simulink model "CEGR_Vehicle_10kW_GZS60_v03_stage2_steadyfit"  (R2025b)
settings: Solver=FixedStepDiscrete  StartTime=0.0  StopTime=120  FixedStep=0.1  RelTol=1e-3
model workspace (MAT data in the model file):
  CompressorParam_v2 = [55; 35]
  EGRInitialNode_v2 = [0; 0; 0; 0; 25; 101.325; 0]
  EnvParam_v2 = [96485.33212; 0.031998; 0.0280134; 0.01801528; 101.325; 25; 0.5; 0.2095; 0.7905; 16; 2]
  HumidifierParam_v2 = [0.031998; 0.0280134; 0.01801528; 101.325; 55; 0.47854; 0.0983333333333; 0.37998; 0.5825; 4.58289; 11.4663; 0.868128; 40; 5e-05; 1e-09; 0.02; 0.02; 80]
  I_stack_cmd_A = 120
  IntercoolerParam_v2 = [0.031998; 0.0280134; 0.01801528; 101.325; 55; 8]
  P_v2.rootDir = 'E:\agentwork_pemfc_cEGR_0519\01_自吸方案\01_车载系统_10kW_GZS60_v3'
  P_v2.inputDir = 'E:\agentwork_pemfc_cEGR_0519\01_自吸方案\01_车载系统_10kW_GZS60_v3\00_输入参数'
  P_v2.modelName = 'CEGR_Vehicle_10kW_GZS60_v03'
  P_v2.modelFile = 'E:\agentwork_pemfc_cEGR_0519\01_自吸方案\01_车载系统_10kW_GZS60_v3\01_模型\CEGR_Vehicle_10kW_GZS60_v03.slx'
  P_v2.stopTime_s = 120
  P_v2.dt_s = 0.1
  P_v2.R_J_molK = 8.314462618
  P_v2.F_C_mol = 96485.33212
  P_v2.M_O2_kg_mol = 0.031998
  P_v2.M_N2_kg_mol = 0.0280134
  P_v2.M_H2O_kg_mol = 0.01801528
  P_v2.M_H2_kg_mol = 0.00201588
  P_v2.p_amb_kPa = 101.325
  P_v2.T_amb_C = 25
  P_v2.RH_amb = 0.5
  P_v2.xO2_dry = 0.2095
  P_v2.xN2_dry = 0.7905
  P_v2.N_cell = 16
  P_v2.A_cell_cm2 = 380
  P_v2.I_stack_default_A = 120
  P_v2.oxygen_stoich = 2
  P_v2.anode_stoich = 1.35
  P_v2.RH_an_in = 0.3
  P_v2.compressor_dp_kPa = 55
  P_v2.compressor_dT_C = 35
  P_v2.intercooler_T_C = 55
  P_v2.intercooler_dp_kPa = 8
  P_v2.p_cathode_back_kPa = 128
  P_v2.p_anode_back_kPa = 85
  P_v2.p_anode_in_kPa = 140
  P_v2.K_ca_in_kg_s_kPa = 0.00135
  P_v2.hum_NTU_ref = 0.47854
  P_v2.hum_m_ref_kg_s = 0.0983333333333
  P_v2.hum_flow_exp = 0.37998
  P_v2.hum_heat_eff = 0.5825
  P_v2.hum_dry_dp_ref_kPa = 4.58289
  P_v2.hum_wet_dp_ref_kPa = 11.4663
  P_v2.hum_dp_exp = 0.868128
  P_v2.hum_mem_area_m2 = 40
  P_v2.hum_mem_thickness_m = 5e-05
  P_v2.hum_mem_D_eff_m2_s = 1e-09
  P_v2.hum_beta_wet_m_s = 0.02
  P_v2.hum_beta_dry_m_s = 0.02
  P_v2.hum_UA_W_K = 80
  P_v2.V_ca_m3 = 0.0025
  P_v2.V_an_m3 = 0.0012
  P_v2.K_ca_out_kg_s_kPa = 0.000216
  P_v2.K_an_out_kg_s_kPa = 6.67e-06
  P_v2.K_liq_carry_1_s = 0.08
  P_v2.C_stack_J_K = 45000
  P_v2.h_cool_W_K = 121
  P_v2.T_cool_C = 62
  P_v2.h_amb_W_K = 9
  P_v2.k_mem_water_kg_s = 0.00012
  P_v2.E_nernst_ref_V = 1.229
  P_v2.E_nernst_temp_coeff_V_K = 0.000845879868025
  P_v2.book_xi1 = -1.18256193785
  P_v2.book_xi2 = 0.00294108739023
  P_v2.book_xi3 = 5.21269240296e-05
  P_v2.book_xi4 = -8.54349163446e-05
  P_v2.membraneThickness_cm = 0.005
  P_v2.book_contact_resistance_ohm = 2.22044867148e-14
  P_v2.book_concentration_m_V = 3.97280101898e-05
  P_v2.book_concentration_n_1_A = 0.00982352283961
  P_v2.thermoneutralVoltage_V = 1.254
  P_v2.LHV_H2_J_mol = 241800
  P_v2.stack_m_act_O2 = 0.65
  P_v2.stack_m_lim_O2 = 1.2
  P_v2.stack_i_lim_ref_A_cm2 = 1.2
  P_v2.stack_lambda_O2_half = 1.2
  P_v2.separator_liq_eff = 0.98
  P_v2.egr_fraction_default = 0.4
  P_v2.separator_dp_ref_kPa = 2
  P_v2.tailgas_manifold_dp_kPa = 0.5
  P_v2.egr_return_target_margin_kPa = 0
  P_v2.V_tailgas_manifold_m3 = 0.003
  P_v2.K_tailgas_egr_out_kg_s_kPa = 4e-05
  P_v2.K_tailgas_bp_out_kg_s_kPa = 0.00012
  P_v2.egr_valve_coeff = 1.2
  P_v2.egr_valve_dp_fraction = 0.65
  P_v2.bp_valve_coeff = 2.8
  P_v2.egr_return_pipe_dp_ref_kPa = 1.5
  P_v2.egr_return_pipe_dp_exp = 1
  P_v2.p_anode_tail_downstream_kPa = 85
  P_v2.V_ca_manifold_m3 = 0.0011
  P_v2.V_an_manifold_m3 = 0.0032
  P_v2.K_ca_man_out_kg_s_kPa = 0.0012
  P_v2.K_an_man_out_kg_s_kPa = 4e-05
  P_v2.EnvParam = [96485.33212; 0.031998; 0.0280134; 0.01801528; 101.325; 25; 0.5; 0.2095; 0.7905; 16; 2]
  P_v2.CompressorParam = [55; 35]
  P_v2.IntercoolerParam = [0.031998; 0.0280134; 0.01801528; 101.325; 55; 8]
  P_v2.HumidifierParam = [0.031998; 0.0280134; 0.01801528; 101.325; 55; 0.47854; 0.0983333333333; 0.37998; 0.5825; 4.58289; 11.4663; 0.868128; 40; 5e-05; 1e-09; 0.02; 0.02; 80]
  P_v2.StackParam = [8.314462618; 96485.33212; 0.031998; 0.0280134; 0.01801528; 0.00201588; 101.325; 25; 16; 380; 0.0025; 0.0012; 0.000216; 6.67e-06; 128; 85; 0.08; 45000; 121; 62; 9; 1.229; 0.000845879868025; -1.18256193785; 0.00294108739023; 5.21269240296e-05; -8.54349163446e-05; 0.005; 2.22044867148e-14; 3.97280101898e-05; 0.00982352283961; 1.254; 1.35; 0.3; 0.1; 0.00012; 140; 0.00135; 0.65; 1.2; 1.2; 1.2; 241800]
  P_v2.SeparatorParam = [0.031998; 0.0280134; 0.01801528; 0.98; 101.325; 2; 0.0983333333333; 0.72344]
  P_v2.TailGasParam = [8.314462618; 0.031998; 0.0280134; 0.01801528; 0.003; 4e-05; 0.00012; 0.08; 0.1; 101.325; 0]
  P_v2.CathodeOutletManifoldParam = [8.314462618; 0.031998; 0.0280134; 0.01801528; 0.0011; 0.0012; 0.08; 0.1; 101.325]
  P_v2.AnodeOutletManifoldParam = [8.314462618; 0.00201588; 0.0280134; 0.01801528; 0.0032; 4e-05; 0.08; 0.1; 101.325]
  P_v2.EGRValveParam = [1.2; 0.65]
  P_v2.BackPressureValveParam = [2.8; 101.325]
  P_v2.EGRReturnPipeParam = [101.325; 1.5; 0.0983333333333; 1]
  P_v2.egr_initial_node = [0; 0; 0; 0; 25; 101.325; 0]
  P_v2.wet_initial_node = [0; 0; 0; 0; 70; 128; 0]
  P_v2.ca_manifold_initial_state = [0.000232010722367; 0.000925320943558; 0.00017649999609; 0]
  P_v2.an_manifold_initial_state = [0.000177788459184; 0; 0.000154036360224; 0]
  P_v2.tailgas_manifold_initial_state = [0.000549996359197; 0.00219353288871; 0.0004813636257; 0]
  P_v2.stack_initial_state = [0.000711310590109; 0.00236638748431; 0.000400476887549; 0; 0.000111852500588; 5.7763635084e-05; 0; 65]
  P_v2.stack_initial_state_audit = [0.000711310590109; 0.00236638748431; 0.000400476887549; 0.000111852500588; 5.7763635084e-05; 65]
  StackInitialStateAudit_v3 = [0.000711310590109; 0.00236638748431; 0.000400476887549; 0.000111852500588; 5.7763635084e-05; 65]
  StackParam_v2 = [8.314462618; 96485.33212; 0.031998; 0.0280134; 0.01801528; 0.00201588; 101.325; 25; 16; 380; 0.0025; 0.0012; 0.000216; 6.67e-06; 128; 85; 0.08; 45000; 121; 62; 9; 1.229; 0.000845879868025; -1.18256193785; 0.00294108739023; 5.21269240296e-05; -8.54349163446e-05; 0.005; 2.22044867148e-14; 3.97280101898e-05; 0.00982352283961; 1.254; 1.35; 0.3; 0.1; 0.00012; 140; 0.00135; 0.65; 1.2; 1.2; 1.2; 241800]
  WetInitialNode_v2 = [0; 0; 0; 0; 70; 128; 0]
  egr_fraction_cmd = 0
settings Model: Creator=ADMIN  LastModifiedBy=ADMIN

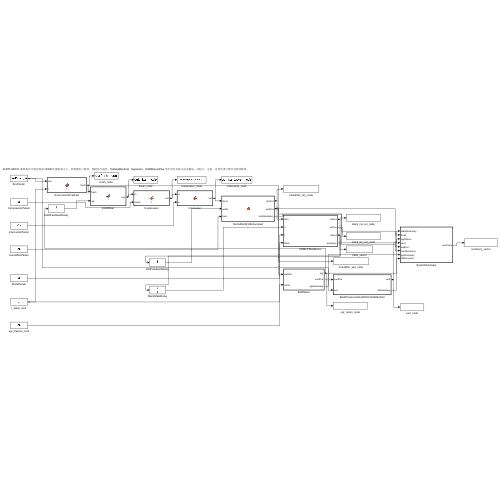
[thumbnail: Simulink's stored preview of the top-level diagram]
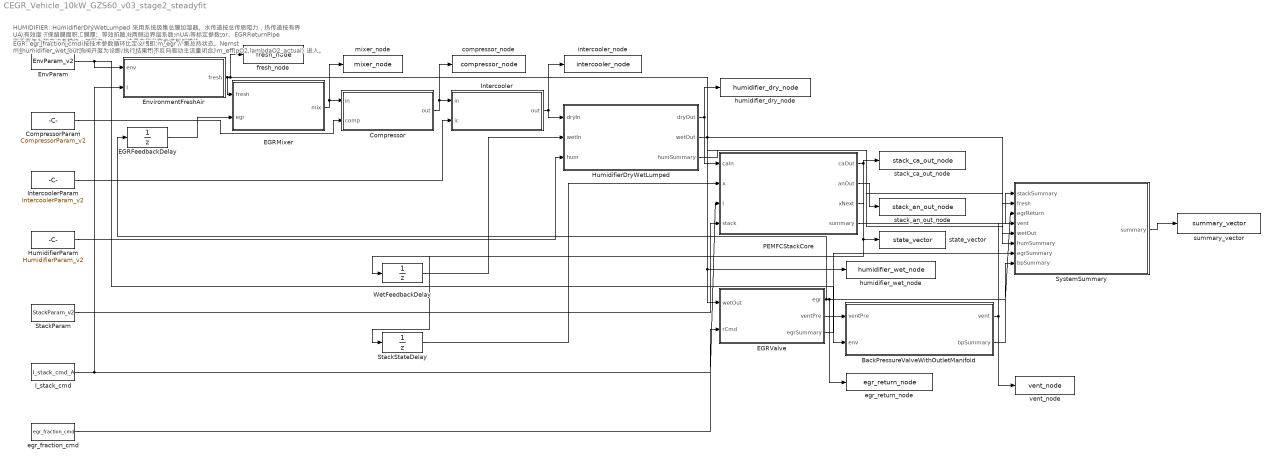
== system CEGR_Vehicle_10kW_GZS60_v03_stage2_steadyfit ==
  note: AUDIT-ARCH: 新架构审计版仅保留 cEGR 性能影响主干。旧阴极出口歧管、阳极尾气歧管、TailGasManifold、Separator、EGRReturnPipe 等不再作为独立动态模块；其阻力、分流、边界作用已整合进相邻模块。
  note: STACK: PEMFCStackCore 使用 5 个气体组分质量状态 + 1 个集总热状态。Nernst 不做经验修改，氧浓度影响通过活化过电势 i0_c_eff(pO2) 和浓差过电势 i_lim_eff(pO2,lambdaO2_actual) 进入。
  note: HUMIDIFIER: HumidifierDryWetLumped 采用系统级集总膜加湿器。水传递按总传质阻力，热传递按有界 UA/有效度，保留膜面积、膜厚、等效扩散、两侧边界层系数、UA 等标定参数。
  note: EGR: egr_fraction_cmd 按技术参数循环比定义，即 m_egr / m_humidifier_wet_out。阀开度为诊断/执行结果，不反向驱动主流量闭合。
  BackPressureValveWithOutletManifold : MATLAB Function  TreatAsAtomicUnit=on
  Compressor : MATLAB Function  TreatAsAtomicUnit=on
  CompressorParam : Constant  Value=CompressorParam_v2
  EGRFeedbackDelay : UnitDelay  InitialCondition=EGRInitialNode_v2  SampleTime=-1  HasFrameUpgradeWarning=on
  EGRMixer : MATLAB Function  TreatAsAtomicUnit=on
  EGRValve : MATLAB Function  TreatAsAtomicUnit=on
  EnvParam : Constant  Value=EnvParam_v2
  EnvironmentFreshAir : MATLAB Function  TreatAsAtomicUnit=on
  HumidifierDryWetLumped : MATLAB Function  TreatAsAtomicUnit=on
  HumidifierParam : Constant  Value=HumidifierParam_v2
  I_stack_cmd : Constant  Value=I_stack_cmd_A
  Intercooler : MATLAB Function  TreatAsAtomicUnit=on
  IntercoolerParam : Constant  Value=IntercoolerParam_v2
  PEMFCStackCore : MATLAB Function  TreatAsAtomicUnit=on
  StackParam : Constant  Value=StackParam_v2
  StackStateDelay : UnitDelay  InitialCondition=StackInitialStateAudit_v3  SampleTime=-1  HasFrameUpgradeWarning=on
  SystemSummary : MATLAB Function  TreatAsAtomicUnit=on
  WetFeedbackDelay : UnitDelay  InitialCondition=WetInitialNode_v2  SampleTime=-1  HasFrameUpgradeWarning=on
  compressor_node : ToWorkspace  VariableName=compressor_node  SampleTime=-1
  egr_fraction_cmd : Constant  Value=egr_fraction_cmd
  egr_return_node : ToWorkspace  VariableName=egr_return_node  SampleTime=-1
  fresh_node : ToWorkspace  VariableName=fresh_node  SampleTime=-1
  humidifier_dry_node : ToWorkspace  VariableName=humidifier_dry_node  SampleTime=-1
  humidifier_wet_node : ToWorkspace  VariableName=humidifier_wet_node  SampleTime=-1
  intercooler_node : ToWorkspace  VariableName=intercooler_node  SampleTime=-1
  mixer_node : ToWorkspace  VariableName=mixer_node  SampleTime=-1
  stack_an_out_node : ToWorkspace  VariableName=stack_an_out_node  SampleTime=-1
  stack_ca_out_node : ToWorkspace  VariableName=stack_ca_out_node  SampleTime=-1
  state_vector : ToWorkspace  VariableName=state_vector  SampleTime=-1
  summary_vector : ToWorkspace  VariableName=summary_vector  SampleTime=-1
  vent_node : ToWorkspace  VariableName=vent_node  SampleTime=-1
  wires:
  EnvParam/1 -> EnvironmentFreshAir/1(env), BackPressureValveWithOutletManifold/2(env)
  I_stack_cmd/1 -> EnvironmentFreshAir/2(I), PEMFCStackCore/3(I)
  EnvironmentFreshAir/1(fresh) -> fresh_node/1, SystemSummary/2(fresh), EGRMixer/1(fresh)
  EGRFeedbackDelay/1 -> EGRMixer/2(egr)
  EGRMixer/1(mix) -> Compressor/1(in), mixer_node/1
  CompressorParam/1 -> Compressor/2(comp)
  Compressor/1(out) -> Intercooler/1(in), compressor_node/1
  IntercoolerParam/1 -> Intercooler/2(ic)
  Intercooler/1(out) -> HumidifierDryWetLumped/1(dryIn), intercooler_node/1
  WetFeedbackDelay/1 -> HumidifierDryWetLumped/2(wetIn)
  HumidifierParam/1 -> HumidifierDryWetLumped/3(hum)
  HumidifierDryWetLumped/1(dryOut) -> PEMFCStackCore/1(caIn), humidifier_dry_node/1
  StackStateDelay/1 -> PEMFCStackCore/2(x)
  StackParam/1 -> PEMFCStackCore/4(stack)
  PEMFCStackCore/1(caOut) -> WetFeedbackDelay/1, stack_ca_out_node/1
  PEMFCStackCore/2(anOut) -> stack_an_out_node/1
  PEMFCStackCore/3(xNext) -> StackStateDelay/1, state_vector/1
  HumidifierDryWetLumped/2(wetOut) -> EGRValve/1(wetOut), humidifier_wet_node/1, SystemSummary/5(wetOut)
  egr_fraction_cmd/1 -> EGRValve/2(rCmd)
  EGRValve/1(egr) -> egr_return_node/1, SystemSummary/3(egrReturn), EGRFeedbackDelay/1
  EGRValve/2(ventPre) -> BackPressureValveWithOutletManifold/1(ventPre)
  BackPressureValveWithOutletManifold/1(vent) -> vent_node/1, SystemSummary/4(vent)
  PEMFCStackCore/4(summary) -> SystemSummary/1(stackSummary)
  HumidifierDryWetLumped/3(humSummary) -> SystemSummary/6(humSummary)
  EGRValve/3(egrSummary) -> SystemSummary/7(egrSummary)
  BackPressureValveWithOutletManifold/2(bpSummary) -> SystemSummary/8(bpSummary)
  SystemSummary/1(summary) -> summary_vector/1

== matlab function CEGR_Vehicle_10kW_GZS60_v03_stage2_steadyfit/EGRMixer ==
  data: fresh input; mix output; egr input
function mix = f(fresh, egr)
%#codegen
% EGR 掺混口径：总进空压机质量流保持新鲜空气基准，回流尾气替代等质量新鲜空气。
mix=zeros(7,1); mf0=max(sum(fresh(1:4)),0); me0=max(sum(egr(1:4)),0); me=min(me0,0.95*mf0); mf=max(mf0-me,0);
wFresh=fresh(1:4)/max(mf0,1e-12); wEgr=egr(1:4)/max(me0,1e-12);
mix(1:4)=mf*wFresh+me*wEgr; mt=max(mf+me,1e-12);
mix(5)=(fresh(5)*mf+egr(5)*me)/mt;
mix(6)=(fresh(6)*mf+egr(6)*me)/mt;
mix(7)=double(mix(4)>1e-12);
end

== matlab function CEGR_Vehicle_10kW_GZS60_v03_stage2_steadyfit/EnvironmentFreshAir ==
  data: env input; fresh output; I input
function fresh = f(env, I)
%#codegen
F=env(1); M_O2=env(2); M_N2=env(3); M_H2O=env(4); pamb=env(5); Tamb=env(6); RH=env(7); xO2=env(8); xN2=env(9); N=env(10); stoich=env(11);
psat=sat_kPa(Tamb); pH2O=min(RH*psat,0.98*pamb); pdry=max(pamb-pH2O,1e-6);
pO2=xO2*pdry; pN2=xN2*pdry;
nO2=stoich*max(I,0)*N/(4*F);
mO2=max(nO2*M_O2,1e-7); scale=(mO2/M_O2)/max(pO2,1e-9);
fresh=[mO2; pN2*scale*M_N2; pH2O*scale*M_H2O; 0; Tamb; pamb; 0];
end
function p=sat_kPa(T)
p=0.61121*exp((18.678-T/234.5)*(T/(257.14+T)));
end

== matlab function CEGR_Vehicle_10kW_GZS60_v03_stage2_steadyfit/Compressor ==
  data: in input; out output; comp input
function out = f(in, comp)
%#codegen
out=in; out(6)=in(6)+comp(1); out(5)=in(5)+comp(2); out(7)=double(out(4)>1e-12);
end

== matlab function CEGR_Vehicle_10kW_GZS60_v03_stage2_steadyfit/Intercooler ==
  data: in input; out output; ic input
function out = f(in, ic)
%#codegen
out=in; M_O2=ic(1); M_N2=ic(2); M_H2O=ic(3); pamb=ic(4); Tout=ic(5); dp=ic(6);
out(5)=Tout; out(6)=max(in(6)-dp,pamb);
ps=min(sat_kPa(Tout),0.98*out(6)); nDry=max(out(1)/M_O2+out(2)/M_N2,1e-12); mSat=ps*nDry/max(out(6)-ps,1e-6)*M_H2O;
if out(3)>mSat, out(4)=out(4)+out(3)-mSat; out(3)=mSat; end
out(7)=double(out(4)>1e-12);
end
function p=sat_kPa(T)
p=0.61121*exp((18.678-T/234.5)*(T/(257.14+T)));
end

== matlab function CEGR_Vehicle_10kW_GZS60_v03_stage2_steadyfit/HumidifierDryWetLumped ==
  data: dryIn input; dryOut output; wetIn input; hum input; wetOut output; humSummary output
function [dryOut, wetOut, humSummary] = f(dryIn, wetIn, hum)
%#codegen
M_O2=hum(1); M_N2=hum(2); M_H2O=hum(3); pamb=hum(4); mRef=max(hum(7),1e-9);
A=hum(13); delta=max(hum(14),1e-9); Deff=max(hum(15),1e-12); betaW=max(hum(16),1e-6); betaD=max(hum(17),1e-6); UA=max(hum(18),0);
mDry=max(sum(dryIn(1:4)),1e-9); mWet=max(sum(wetIn(1:4)),1e-9);
pD=vapor_p(dryIn,M_O2,M_N2,M_H2O); pW=vapor_p(wetIn,M_O2,M_N2,M_H2O);
Rtot=1/betaW+delta/Deff+1/betaD;
j=max((pW-pD)*1000,0)/(8.314462618*max(dryIn(5)+273.15,250)*Rtot);
mTransRaw=j*A*M_H2O; dryNeed=max(vapor_sat_mass(dryIn(1),dryIn(2),dryIn(5),dryIn(6),hum)-dryIn(3),0); wetAvail=max(wetIn(3),0);
mTrans=min([mTransRaw,dryNeed,wetAvail]);
Cmin=max(min(mDry,mWet)*1050,1e-6); epsH=min(max(1-exp(-UA/Cmin),0),0.85); dTDry=min(max(epsH*(wetIn(5)-dryIn(5))*Cmin/(mDry*1050),-30),30);
dryOut=dryIn; dryOut(3)=dryIn(3)+mTrans; dryOut(5)=min(max(dryIn(5)+dTDry,-20),95);
dpDry=hum(10)*(mDry/mRef)^hum(12); dryOut(6)=max(dryIn(6)-dpDry,pamb);
[dryOut(3),dryOut(4)]=clip_vapor(dryOut(3),dryOut(4),dryOut(1),dryOut(2),dryOut(5),dryOut(6),hum); dryOut(7)=double(dryOut(4)>1e-12);
wetOut=wetIn; wetOut(3)=max(wetIn(3)-mTrans,0); wetOut(5)=min(max(wetIn(5)-dTDry,-20),95);
dpWet=hum(11)*(mWet/mRef)^hum(12); wetOut(6)=max(wetIn(6)-dpWet,pamb);
[wetOut(3),wetOut(4)]=clip_vapor(wetOut(3),wetOut(4),wetOut(1),wetOut(2),wetOut(5),wetOut(6),hum); wetOut(7)=double(wetOut(4)>1e-12);
humSummary=[mTrans; mTransRaw; pW-pD; dTDry; dpDry; dpWet; rel_hum(dryOut,M_O2,M_N2,M_H2O); rel_hum(wetOut,M_O2,M_N2,M_H2O)];
end
function p=vapor_p(node,M_O2,M_N2,M_H2O)
nV=max(node(3)/M_H2O,0); nt=max(node(1)/M_O2+node(2)/M_N2+nV,1e-12); p=node(6)*nV/nt;
end
function rh=rel_hum(node,M_O2,M_N2,M_H2O)
rh=vapor_p(node,M_O2,M_N2,M_H2O)/max(sat_kPa(node(5)),1e-6);
end
function mSat=vapor_sat_mass(mO2,mN2,T,p,hum)
M_O2=hum(1); M_N2=hum(2); M_H2O=hum(3); ps=min(sat_kPa(T),0.98*p); nDry=max(mO2/M_O2+mN2/M_N2,1e-12); mSat=ps*nDry/max(p-ps,1e-6)*M_H2O;
end
function [mv,ml]=clip_vapor(mv0,ml0,mO2,mN2,T,p,hum)
mSat=vapor_sat_mass(mO2,mN2,T,p,hum); if mv0>mSat, mv=mSat; ml=ml0+mv0-mSat; else, mv=mv0; ml=ml0; end
end
function p=sat_kPa(T)
Tc=min(max(T,-40),120); p=0.61121*exp((18.678-Tc/234.5)*(Tc/(257.14+Tc)));
end

== matlab function CEGR_Vehicle_10kW_GZS60_v03_stage2_steadyfit/PEMFCStackCore ==
  data: caIn input; caOut output; x input; I input; stack input; anOut output; xNext output; summary output
function [caOut, anOut, xNext, summary] = f(caIn, x, I, stack)
%#codegen
R=stack(1); F=stack(2); M_O2=stack(3); M_N2=stack(4); M_H2O=stack(5); M_H2=stack(6); pamb=stack(7); Tamb=stack(8); N=stack(9); A=stack(10);
Vca=stack(11); Van=stack(12); Kca=stack(13); Kan=stack(14); pcBack=stack(15); panBack=stack(16); Cfc=stack(18); hCool=stack(19); Tcool=stack(20); hAmb=stack(21);
Eref=stack(22); Etemp=stack(23); xi1=stack(24); xi2=stack(25); xi3=stack(26); xi4=stack(27); deltaCm=stack(28); rContact=stack(29); concM=stack(30); anStoich=stack(33); RHAn=stack(34); dt=stack(35); panIn=stack(37); KcaIn=stack(38); mAct=stack(39); mLim=stack(40); iLimRef=stack(41); lambdaHalf=stack(42); LHV=stack(43);
mO2=max(x(1),1e-12); mN2=max(x(2),1e-12); mV=max(x(3),0); mH2=max(x(4),1e-12); mVAn=max(x(5),0); T=x(6); TK=T+273.15;
pO2=mO2/M_O2*R*TK/Vca/1000; pN2=mN2/M_N2*R*TK/Vca/1000; pV=mV/M_H2O*R*TK/Vca/1000; pCa=max(pO2+pN2+pV,pamb);
pVAn=mVAn/M_H2O*R*TK/Van/1000;
mInCmd=sum(caIn(1:3)); mInPressure=KcaIn*max(caIn(6)-pCa,0); mIn=min(mInCmd,mInPressure); wIn=caIn(1:3)/max(mInCmd,1e-12); mO2In=mIn*wIn(1); mN2In=mIn*wIn(2); mVIn=mIn*wIn(3);
mO2React=I*N/(4*F)*M_O2; mH2React=I*N/(2*F)*M_H2; mWater=I*N/(2*F)*M_H2O; lambdaO2=(mO2In/M_O2)/max(I*N/(4*F),1e-12);
ps=sat_kPa(T); aCa=min(max(pV/max(ps,1e-6),0),3); aAn=min(max(pVAn/max(ps,1e-6),0),3); lam=0.5*(lambda_eq(aCa)+lambda_eq(aAn));
A_m2=A*1e-4; nDrag=max(0.0029*lam^2+0.05*lam,0); D=membrane_diff(lam,TK); cCa=pV*1000/(R*TK); cAn=pVAn*1000/(R*TK); mMem=(nDrag*I/F - D*A_m2*N/max(deltaCm*0.01,1e-9)*(cCa-cAn))*M_H2O;
mH2In=anStoich*mH2React; pH2OIn=RHAn*ps; mVAnIn=mH2In*max(pH2OIn,0)/max(panIn-pH2OIn,1e-6)*(M_H2O/M_H2);
mO2Pre=max(mO2+dt*(mO2In-mO2React),1e-12); mN2Pre=max(mN2+dt*mN2In,1e-12); mVPre=max(mV+dt*(mVIn+mWater+mMem),0);
mH2Pre=max(mH2+dt*(mH2In-mH2React),1e-12); mVAnPre=max(mVAn+dt*(mVAnIn-mMem),0);
pO2Pre=mO2Pre/M_O2*R*TK/Vca/1000; pN2Pre=mN2Pre/M_N2*R*TK/Vca/1000; pVPre=mVPre/M_H2O*R*TK/Vca/1000; pCaPre=max(pO2Pre+pN2Pre+pVPre,pamb);
pH2Pre=mH2Pre/M_H2*R*TK/Van/1000; pVAnPre=mVAnPre/M_H2O*R*TK/Van/1000; pAnPre=max(pH2Pre+pVAnPre,pamb);
gasCa=max(mO2Pre+mN2Pre+mVPre,1e-12); mCaOut=min(Kca*max(pCaPre-pcBack,0),0.8*gasCa/max(dt,1e-9)); wO2=mO2Pre/gasCa; wN2=mN2Pre/gasCa; wV=mVPre/gasCa;
gasAn=max(mH2Pre+mVAnPre,1e-12); mAnOut=min(Kan*max(pAnPre-panBack,0),0.8*gasAn/max(dt,1e-9)); wH2=mH2Pre/gasAn; wVAn=mVAnPre/gasAn;
mO2n=max(mO2Pre-dt*wO2*mCaOut,1e-12); mN2n=max(mN2Pre-dt*wN2*mCaOut,1e-12); mVnRaw=max(mVPre-dt*wV*mCaOut,0);
mH2n=max(mH2Pre-dt*wH2*mAnOut,1e-12); mVAnnRaw=max(mVAnPre-dt*wVAn*mAnOut,0);
[mVn,liqDiag]=clip_vapor(mVnRaw,0,mO2n,mN2n,T,pCaPre,stack,0); [mVAnn,liqAnDiag]=clip_vapor(mVAnnRaw,0,mH2n,0,T,pAnPre,stack,1);
phaseCa=(mVnRaw-mVn)/dt; phaseAn=(mVAnnRaw-mVAnn)/dt;
j=max(I/max(A,1e-9),1e-6); pO2r=max(pO2Pre,1e-6)/21.0; E=Eref-Etemp*(TK-298.15)+R*TK/(2*F)*log(max(pH2Pre*1000,1)/101325*sqrt(max(pO2Pre*1000,1)/101325));
CO2=max((pO2Pre*1000)/(5.08e6*exp(-498/TK)),1e-12); i0Scale=max(pO2r^mAct,0.05); etaAct=max(-(xi1+xi2*TK+xi3*TK*log(CO2*i0Scale)+xi4*TK*log(max(I,1e-6))),0);
sigma=max((0.005139*max(lam,1)-0.00326)*exp(1268*(1/303.15-1/TK)),0.02); etaOhm=I*(deltaCm/sigma/max(A,1e-9)+rContact);
flowFactor=lambdaO2/max(lambdaO2+lambdaHalf,1e-9); iLim=max(iLimRef*(max(pO2r,0.02)^mLim)*flowFactor,j+0.02); etaCon=max(concM*log(1/max(1-j/iLim,1e-4)),0);
V=max(E-etaAct-etaOhm-etaCon,0.2); Pstack=I*V*N; Qgen=I*N*LHV/(2*F)-Pstack; Qcool=hCool*(T-Tcool); Qamb=hAmb*(T-Tamb); Qgas=max(mCaOut+mAnOut,0)*1050*max(T-caIn(5),0); Qnet=Qgen-Qcool-Qamb-Qgas; Tn=T+dt*Qnet/Cfc;
xNext=[mO2n;mN2n;mVn;mH2n;mVAnn;Tn]; caOut=[wO2*mCaOut;wN2*mCaOut;wV*mCaOut;0;Tn+3;pCaPre;0]; anOut=[wH2*mAnOut;0;wVAn*mAnOut;0;Tn;pAnPre;0];
nTot=max(mO2n/M_O2+mN2n/M_N2+mVn/M_H2O,1e-12); xO2=(mO2n/M_O2)/nTot; RH=(mVn/M_H2O*R*(Tn+273.15)/Vca/1000)/max(sat_kPa(Tn),1e-6);
nInTot=max(caIn(1)/M_O2+caIn(2)/M_N2+caIn(3)/M_H2O,1e-12); xO2In=(caIn(1)/M_O2)/nInTot; pO2In=caIn(6)*xO2In; RHIn=(caIn(6)*(caIn(3)/M_H2O)/nInTot)/max(sat_kPa(caIn(5)),1e-6);
resO2=(mO2n-mO2)/dt-(mO2In-wO2*mCaOut-mO2React); resN2=(mN2n-mN2)/dt-(mN2In-wN2*mCaOut);
resH2Ov=(mVn-mV)/dt-(mVIn-wV*mCaOut+mWater+mMem-phaseCa);
resH2=(mH2n-mH2)/dt-(mH2In-wH2*mAnOut-mH2React); resH2OvAn=(mVAnn-mVAn)/dt-(mVAnIn-wVAn*mAnOut-mMem-phaseAn);
maxGasRes=max(abs([resO2,resN2,resH2Ov,resH2,resH2OvAn]));
summary=[I;V;Pstack;pO2Pre;pCaPre;pH2Pre;pAnPre;lam;Tn;xO2;RH;mMem;mO2React;mH2React;mWater;mCaOut;mAnOut;Cfc*(Tn-T)/dt-Qnet;pO2In;xO2In;RHIn;Qnet;resO2;resN2;resH2Ov;phaseCa;resH2;resH2OvAn;phaseAn;phaseCa+phaseAn;maxGasRes;Qgen;Qcool;Qamb;Qgas;E;etaAct;etaOhm;etaCon;lambdaO2;mIn;iLim;i0Scale;mVIn;wV*mCaOut;mVAnIn;wVAn*mAnOut;liqDiag+liqAnDiag];
end
function [mv,ml]=clip_vapor(mv0,ml0,mA,mB,T,p,stack,isAnode)
M_O2=stack(3); M_N2=stack(4); M_H2O=stack(5); M_H2=stack(6); MA=M_O2; MB=M_N2; if isAnode>0.5, MA=M_H2; end; ps=min(sat_kPa(T),0.98*p); nDry=max(mA/MA+mB/MB,1e-12); mSat=max(ps*nDry/max(p-ps,1e-6)*M_H2O,0); if mv0>mSat, mv=mSat; ml=ml0+mv0-mSat; else, mv=mv0; ml=ml0; end
end
function p=sat_kPa(T)
Tc=min(max(T,-40),120); p=0.61121*exp((18.678-Tc/234.5)*(Tc/(257.14+Tc)));
end
function lambda=lambda_eq(a)
if a<=1, lambda=0.043+17.81*a-39.85*a^2+36*a^3; else, lambda=14+1.4*(a-1); end
end
function D=membrane_diff(lambda,TK)
if lambda<2, d0=1e-10; elseif lambda<3, d0=1e-10*(1+2*(lambda-2)); elseif lambda<4.5, d0=1e-10*(3-1.167*(lambda-3)); else, d0=1.25e-10; end; D=d0*exp(2416*(1/303-1/max(TK,1)));
end

== matlab function CEGR_Vehicle_10kW_GZS60_v03_stage2_steadyfit/EGRValve ==
  data: wetOut input; egr output; rCmd input; ventPre output; egrSummary output
function [egr, ventPre, egrSummary] = f(wetOut, rCmd)
%#codegen
r=min(max(rCmd,0),0.95);
egr=wetOut; egr(1:3)=r*wetOut(1:3); egr(4)=0; egr(7)=0;
ventPre=wetOut; ventPre(1:3)=(1-r)*wetOut(1:3); ventPre(7)=double(ventPre(4)>1e-12);
mWet=sum(wetOut(1:3)); egrSummary=[r; sum(egr(1:3)); sum(ventPre(1:3)); mWet];
end

== matlab function CEGR_Vehicle_10kW_GZS60_v03_stage2_steadyfit/BackPressureValveWithOutletManifold ==
  data: ventPre input; vent output; env input; bpSummary output
function [vent, bpSummary] = f(ventPre, env)
%#codegen
pamb=env(5);
vent=ventPre; dp=max(ventPre(6)-pamb,0); vent(6)=pamb;
bpSummary=[dp; sum(vent(1:3)); pamb];
end

== matlab function CEGR_Vehicle_10kW_GZS60_v03_stage2_steadyfit/SystemSummary ==
  data: stackSummary input; summary output; fresh input; egrReturn input; vent input; wetOut input; humSummary input; egrSummary input; bpSummary input
function summary = f(stackSummary, fresh, egrReturn, vent, wetOut, humSummary, egrSummary, bpSummary)
%#codegen
summary=[stackSummary;sum(fresh(1:3));sum(egrReturn(1:3));sum(vent(1:3));wetOut(6);egrSummary(1);humSummary(1);humSummary(7);humSummary(8);bpSummary(1);humSummary(5);humSummary(6);egrSummary(4);egrSummary(2);egrSummary(3);bpSummary(3)];
end
